simulink model "ejercicio_05_10_jevg"  (R2021a)
settings: Solver=VariableStepAuto  StartTime=0.0  StopTime=10.0  RelTol=1e-3
libraries: fl_lib x13, nesl_utility x5
settings Model: Creator=gandh  LastModifiedBy=user
settings DebuggingCC: UnconnectedInputMsg=none  UnconnectedOutputMsg=none  UnconnectedLineMsg=none
settings ModelReferenceCC: EnableRefExpFcnMdlSchedulingChecks=off
settings RTWCC: Description=Generic Real-Time Target  DLArmComputeVersion=20.02.1

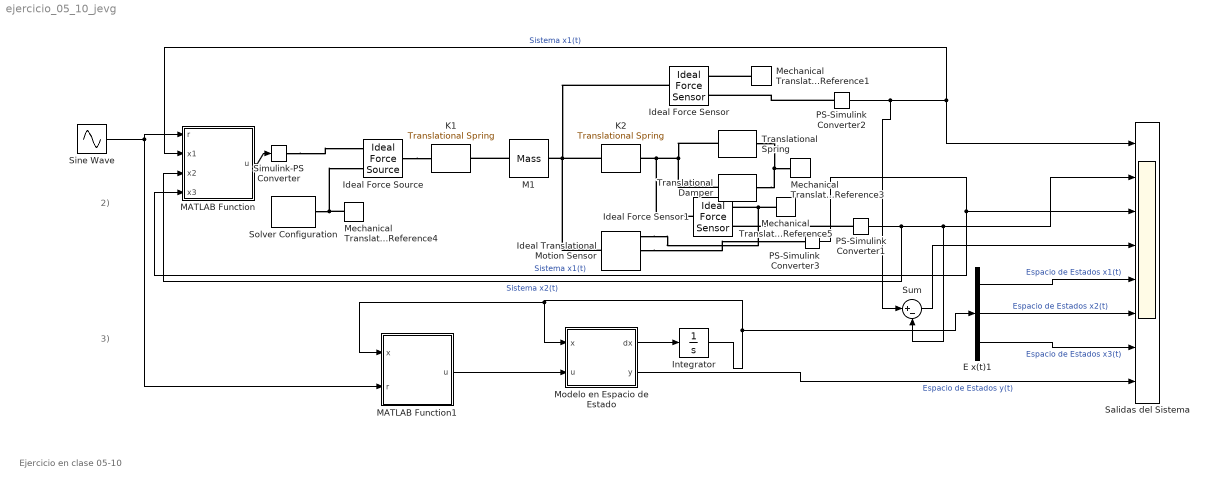
== system ejercicio_05_10_jevg ==
  note: Ejercicio en clase
      | 05-10
  note: 2)
  note: 3)
  E x(t)1 : Demux  Outputs=3
  Ideal Force Sensor : fl_lib/Mechanical/Mechanical Sensors/Ideal Force Sensor
  Ideal Force Sensor1 : fl_lib/Mechanical/Mechanical Sensors/Ideal Force Sensor
  Ideal Force Source : fl_lib/Mechanical/Mechanical Sources/Ideal Force Source
  Ideal Translational Motion Sensor : fl_lib/Mechanical/Mechanical Sensors/Ideal Translational Motion Sensor  offset=0 m
  Integrator : Integrator  InitialCondition=[0 0 0]'
  K1 : fl_lib/Mechanical/Translational Elements/Translational Spring  spr_rate=2 N/m  v_specify=off  v_priority=None  v=0 m/s  v_nominal_specify=off  v_nominal_unit=m/s  v_nominal_value=1  f_specify=off  f_priority=None  f=0 N  f_nominal_specify=off  f_nominal_unit=N  f_nominal_value=1  x_specify=off  x_priority=High  x=0 m  x_nominal_specify=off  x_nominal_unit=m  x_nominal_value=1
  K2 : fl_lib/Mechanical/Translational Elements/Translational Spring  spr_rate=1 N/m  v_specify=off  v_priority=None  v=0 m/s  v_nominal_specify=off  v_nominal_unit=m/s  v_nominal_value=1  f_specify=off  f_priority=None  f=0 N  f_nominal_specify=off  f_nominal_unit=N  f_nominal_value=1  x_specify=off  x_priority=High  x=0 m  x_nominal_specify=off  x_nominal_unit=m  x_nominal_value=1
  M1 : fl_lib/Mechanical/Translational Elements/Mass  mass=10 kg  num_ports=foundation.enum.numPorts2.two  v_specify=off  v_priority=High  v=0 m/s  v_nominal_specify=off  v_nominal_unit=m/s  v_nominal_value=1  f_specify=off  f_priority=None  f=0 N  f_nominal_specify=off  f_nominal_unit=N  f_nominal_value=1
      settings: InternalSimscapePortConfiguration="{\"Bottom\":[],\"Left\":[{\"id\":\"M\",\"label\":\"\",\"type\":\"foundation.mechanical.translational.translational\"}],\"Right\":[{\"id\":\"N\",\"label\":\"\",\"type\":\"foundation.mechanical.translational.translational\"}],\"Top\":[]}"
  MATLAB Function : MATLAB Function  TreatAsAtomicUnit=on
  MATLAB Function1 : MATLAB Function  TreatAsAtomicUnit=on
  Mechanical Translational Reference{1,3..5} (4 alike) : fl_lib/Mechanical/Translational Elements/Mechanical Translational Reference
  Modelo en Espacio de Estado : MATLAB Function  TreatAsAtomicUnit=on
  PS-Simulink Converter1 : nesl_utility/PS-Simulink Converter  PhysicalDomain=network_engine_domain  SubClassName=ps_output  LeftPortType=input  RightPortType=output  PseudoPeriodic=off  Frequencies=[]  Unit=inherit  AffineConversion=off
      settings: SourceProductBaseCode=PW,SS
  PS-Simulink Converter2 : nesl_utility/PS-Simulink Converter  PhysicalDomain=network_engine_domain  SubClassName=ps_output  LeftPortType=input  RightPortType=output  PseudoPeriodic=off  Frequencies=[]  Unit=inherit  AffineConversion=off
      settings: SourceProductBaseCode=PW,SS
  PS-Simulink Converter3 : nesl_utility/PS-Simulink Converter  PhysicalDomain=network_engine_domain  SubClassName=ps_output  LeftPortType=input  RightPortType=output  PseudoPeriodic=off  Frequencies=[]  Unit=inherit  AffineConversion=off
      settings: SourceProductBaseCode=PW,SS
  Salidas del Sistema : Scope  NumInputPorts=8
  Simulink-PS Converter : nesl_utility/Simulink-PS Converter  PhysicalDomain=network_engine_domain  SubClassName=ps_input  LeftPortType=input  RightPortType=output  PseudoPeriodic=off  Frequencies=[]  NoiseDistribution=none  NoiseParameters=[]  Unit=1  AffineConversion=off  FilteringAndDerivatives=filter  SimscapeFilterOrder=1  InputFilterTimeConstant=0.001  UdotUserProvided=0
      settings: SourceProductBaseCode=PW,SS
  Sine Wave : Sin  SampleTime=0
  Solver Configuration : nesl_utility/Solver Configuration  PhysicalDomain=network_engine_domain  SubClassName=solver  LeftPortType=input  RightPortType=generic  Tones=[]  Harmonics=[]  SimulateNoise=off  Profile=off  UseLocalSampling=off  EnableSwitchedLinearOptims=on  FrequencyDomain=off  UseCCode=off  RelTol=0.001  AbsTol=1e-06  MinStep=1e-09  ToWorkspace=off  RevertToSquareIcSolve=off  NumHomotopyIterations=100  PhasorMode=off  PhasorModeNumHarmonics=1  DoDC=off  ResidualTolerance=1e-09  UseLocalSolver=off  LocalSolverChoice=NE_BACKWARD_EULER_ADVANCER  LocalSolverSampleTime=0.001  DoFixedCost=off  MaxNonlinIter=3  MaxModeIter=2  ComputeImpulses=off  ImpulseIterations=2  LinearAlgebra=auto  EquationFormulation=NE_TIME_EF  DelaysMemoryBudget=1024  AutomaticFiltering=on  FilteringTimeConstant=0.001  PartitionStorageMethod=AS_NEEDED  PartitionMemoryBudget=1024  PartitionMethod=ROBUST
      settings: SourceProductBaseCode=PW,SS
  Sum : Sum  Inputs=|+-
  Translational Damper : fl_lib/Mechanical/Translational Elements/Translational Damper  D=0.5 N/(m/s)  v_specify=off  v_priority=None  v=0 m/s  v_nominal_specify=off  v_nominal_unit=m/s  v_nominal_value=1  f_specify=off  f_priority=None  f=0 N  f_nominal_specify=off  f_nominal_unit=N  f_nominal_value=1
  Translational Spring : fl_lib/Mechanical/Translational Elements/Translational Spring  spr_rate=0.50 N/m  v_specify=off  v_priority=None  v=0 m/s  v_nominal_specify=off  v_nominal_unit=m/s  v_nominal_value=1  f_specify=off  f_priority=None  f=0 N  f_nominal_specify=off  f_nominal_unit=N  f_nominal_value=1  x_specify=off  x_priority=High  x=0 m  x_nominal_specify=off  x_nominal_unit=m  x_nominal_value=1
  wires:
  MATLAB Function/1(u) -> Simulink-PS Converter/1
  Sine Wave/1 -> MATLAB Function1/2(r), MATLAB Function/1(r)
  PS-Simulink Converter1/1 -> MATLAB Function/3(x2), Salidas del Sistema/2, Sum/2  "Sistema x2(t)"
  PS-Simulink Converter2/1 -> Salidas del Sistema/1, MATLAB Function/2(x1), Sum/1  "Sistema x1(t)"
  Sum/1 -> Salidas del Sistema/4
  MATLAB Function1/1(u) -> Modelo en Espacio de Estado/2(u)
  Modelo en Espacio de Estado/1(dx) -> Integrator/1
  Integrator/1 -> E x(t)1/1, MATLAB Function1/1(x), Modelo en Espacio de Estado/1(x)
  Modelo en Espacio de Estado/2(y) -> Salidas del Sistema/8  "Espacio de Estados y(t)"
  PS-Simulink Converter3/1 -> MATLAB Function/4(x3), Salidas del Sistema/3  "Sistema x1(t)"
  E x(t)1/1 -> Salidas del Sistema/5  "Espacio de Estados x1(t)"
  E x(t)1/2 -> Salidas del Sistema/6  "Espacio de Estados x2(t)"
  E x(t)1/3 -> Salidas del Sistema/7  "Espacio de Estados x3(t)"
  connections:
  M1/RConn1 -- K1/RConn1
  K2/LConn1 -- Ideal Force Sensor/LConn1 -- Ideal Translational Motion Sensor/LConn1 -- M1/LConn1
  Translational Damper/LConn1 -- Translational Spring/LConn1 -- Ideal Force Sensor1/LConn1 -- K2/RConn1
  Translational Spring/RConn1 -- Mechanical Translational Reference3/LConn1 -- Translational Damper/RConn1
  Mechanical Translational Reference4/LConn1 -- Solver Configuration/RConn1 -- Ideal Force Source/RConn2
  Simulink-PS Converter/RConn1 -- Ideal Force Source/RConn1
  Ideal Force Source/LConn1 -- K1/LConn1
  Mechanical Translational Reference1/LConn1 -- Ideal Force Sensor/RConn1
  Mechanical Translational Reference5/LConn1 -- Ideal Translational Motion Sensor/RConn1 -- Ideal Force Sensor1/RConn1
  PS-Simulink Converter2/LConn1 -- Ideal Force Sensor/RConn2
  PS-Simulink Converter1/LConn1 -- Ideal Force Sensor1/RConn2
  Ideal Translational Motion Sensor/RConn2 -- PS-Simulink Converter3/LConn1

== matlab function ejercicio_05_10_jevg/Modelo en Espacio de Estado ==
  data: x input; dx output; u input; y output
function [dx,y] = fcn(x,u)
% Esta función calcula la derivada del estado dx y la salida y basado en el estado actual x y la señal de control u.

% Definiendo constantes y parámetros del sistema
m1 = 10;
k1 = 2;
k2 = 1;
k3 = 0.5;
b1 = 0.5;

% Definiendo la matriz A del sistema en el espacio de estados
A = [0 1 0; 
    -(k1+k2)/m1 0 k2/m1; 
    k2/b1 0 -(k2+k3)/b1];
% Definiendo la matriz B del sistema en el espacio de estados
B = [0; 
    1/m1; 
    0];

% Definiendo la matriz C para la salida
C=[1 0 -1];

% Calculando la derivada del estado
dx = A*x + B*u;

% Calculando la salida
y = C*x;

== matlab function ejercicio_05_10_jevg/MATLAB Function ==
  data: r input; u output; x1 input; x2 input; x3 input
function u = fcn(r,x1,x2,x3)
% Esta función calcula el control u basado en la entrada r y el estado actual del sistema x.

% Definiendo la matriz de ganancias K
K = [127 39 1];

% Organizando las variables de estado en un vector columna
x = [x1,x2,x3]';

% Calculando la señal de control u usando la retroalimentación de estado
u = r - K*x;

== matlab function ejercicio_05_10_jevg/MATLAB Function1 ==
  data: x input; r input; u output
function u = fcn(x,r)
% Esta función calcula el control u basado en la entrada r y el estado actual del sistema x (como vector).

% Definiendo la matriz de ganancias K
K = [127 39 1];

% Calculando la señal de control u usando la retroalimentación de estado
u = r - K*x;
